simulink model "Es1_S"  (R2014a)
settings: Solver=ode45  StartTime=0.0  StopTime=200  RelTol=1e-3
values from neighbouring files (symbols this model uses):
  Kr = 1    [E1.m]
libraries: cstblocks x3
settings Model: Creator=Davide  LastModifiedBy=Davide

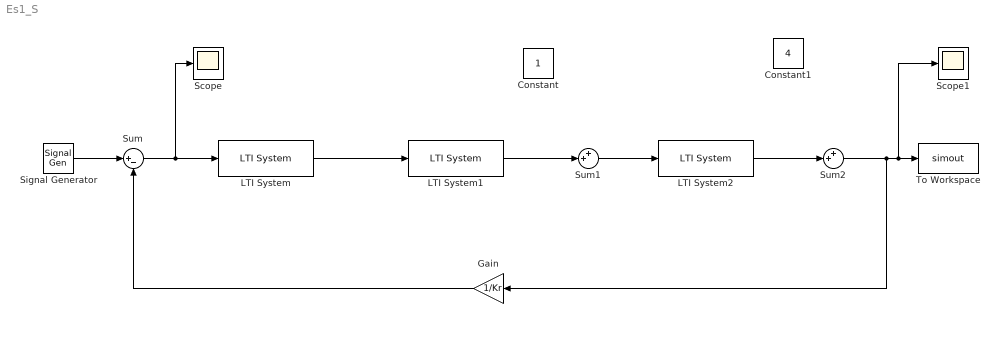
== system Es1_S ==
  Constant : Constant
  Constant1 : Constant  Value=4
  Gain : Gain  Gain=1/Kr
  LTI System : cstblocks/LTI System  sys=C  IC=[]
  LTI System1 : cstblocks/LTI System  sys=F1  IC=[]
  LTI System2 : cstblocks/LTI System  sys=F2  IC=[]
  Scope : Scope
      settings: TimeRange=1.17541766109785  YMin=-0.0169311377245509  YMax=-0.008398203592814367
  Scope1 : Scope
  Signal Generator : SignalGenerator  Frequency=0.2  Units=rad/sec
  Sum : Sum  Inputs=|+-
  Sum1 : Sum  Inputs=++|
  Sum2 : Sum  Inputs=++|
  To Workspace : ToWorkspace  VariableName=simout  SaveFormat=Timeseries  SampleTime=-1
  wires:
  Sum/1 -> Scope/1, LTI System/1
  LTI System/1 -> LTI System1/1
  LTI System1/1 -> Sum1/2
  Sum1/1 -> LTI System2/1
  LTI System2/1 -> Sum2/2
  Sum2/1 -> Gain/1, Scope1/1, To Workspace/1
  Gain/1 -> Sum/2
  Signal Generator/1 -> Sum/1
